simulink model "run_sim"  (R2017a)
settings: Solver=VariableStepAuto  StartTime=0.0  StopTime=10.0  RelTol=1e-3
model workspace: external: MAT-File R:\ggdrive\code\Matlab\QuadSim\Simulink\parameters\param.mat (data not in the file)
settings Model: Creator=calvin  LastModifiedBy=calvin

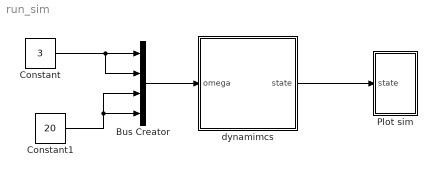
== system run_sim ==
  Bus Creator : BusCreator  Inputs=4
  Constant : Constant  Value=3
  Constant1 : Constant  Value=20
  Plot sim : Subsystem
  dynamimcs : Subsystem
  wires:
  dynamimcs/1(state) -> Plot sim/1(state)
  Bus Creator/1 -> dynamimcs/1(omega)
  Constant/1 -> Bus Creator/2, Bus Creator/1
  Constant1/1 -> Bus Creator/4, Bus Creator/3

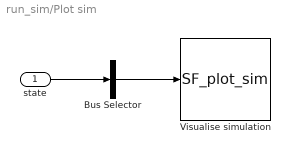
== system run_sim/Plot sim ==
  state : Inport
  Bus Selector : BusSelector  OutputSignals=X,Y,Z,phi,the,psi  OutputAsBus=on
  Visualise simulation : M-S-Function  FunctionName=SF_plot_sim  Parameters=quad
  wires:
  Bus Selector/1 -> Visualise simulation/1
  state/1 -> Bus Selector/1

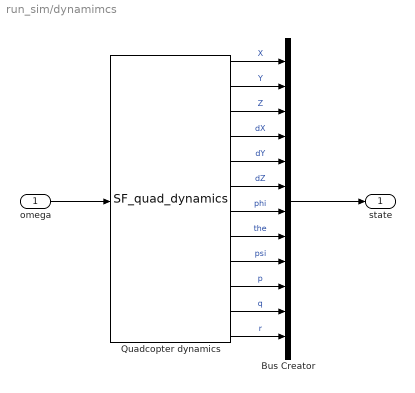
== system run_sim/dynamimcs ==
  omega : Inport
  Bus Creator : BusCreator  Inputs=12
  Quadcopter dynamics : M-S-Function  FunctionName=SF_quad_dynamics  Parameters=quad, x0
  state : Outport
  wires:
  Quadcopter dynamics/10 -> Bus Creator/10  "p"
  Quadcopter dynamics/6 -> Bus Creator/6  "dZ"
  Quadcopter dynamics/2 -> Bus Creator/2  "Y"
  Quadcopter dynamics/4 -> Bus Creator/4  "dX"
  Quadcopter dynamics/3 -> Bus Creator/3  "Z"
  Bus Creator/1 -> state/1
  Quadcopter dynamics/7 -> Bus Creator/7  "phi"
  Quadcopter dynamics/8 -> Bus Creator/8  "the"
  Quadcopter dynamics/12 -> Bus Creator/12  "r"
  Quadcopter dynamics/9 -> Bus Creator/9  "psi"
  omega/1 -> Quadcopter dynamics/1
  Quadcopter dynamics/1 -> Bus Creator/1  "X"
  Quadcopter dynamics/5 -> Bus Creator/5  "dY"
  Quadcopter dynamics/11 -> Bus Creator/11  "q"
